simulink model "ALGO_Corner_Tanker_and_SP"  (Simulink 9.3)
settings: Solver=VariableStepAuto  StartTime=0  StopTime=15  RelTol=1e-3
libraries: simulink x22, Solver_SF x1
(part 2 of 2)

== matlab function 5DOF牵引车半挂车模型 50%液体 单摆模拟/TrailorTruck_5DOF_SP_50per ==
  data: vx input double; state output double; delta input double; observe output double
function [state,observe]=TrailorTruck_5DOF_SP(vx,delta)
%% 初始状态定义
%要记得设置本模块的采样时间哦
persistent Ts                             %采样时间    
persistent state0                         %上一时刻状态
if isempty(state0)
   Ts=0.01;%采样时间
   %初始化状态量
   vx10=vx(1);vx20=vx(2);
   vy10=0; df10=0;F10=0;dF10=0; Y10=0;X10=0;f10=0; %牵引车状态变量
   vy20=0; df20=0;F20=0;dF20=0; Y20=0;X20=-5.638315;f20=0;%半挂车状态变量
   th0=0; dth0=0;%等效摆状态变量
   state0=[vy10,df10,F10,dF10,vy20,df20,F20,dF20,...
       th0,dth0,f10,f20,vx10,vx20,Y10,X10,Y20,X20]';
   
end
%% 定义动力学模型参数
persistent a b c d e                    %轴距纵向几何参数
persistent Tw1 Tw2                      %轮距横向几何参数
persistent h1 h2 hc1 hc2                %质心至侧倾轴线距离
                                        %铰接点至侧倾轴线距离
persistent m1 m2 m1s m2s g;g=9.806;
persistent I1zz I1xx I1xz I2zz I2xx I2xz %惯性参量
persistent k1 k2 k3                      %线性轮胎模型参数
persistent kr1 kr2 c1 c2 k12             %悬架模型参数
persistent m0 mp h0 hp lp co             %等效摆模型参数
if isempty(a)
%摆模型参数
x=[10890,1.5,0.13,0.97,0.13];
sim_param=getParam_SP(x);
% sim_param=[m0,m1,h0+0.77,hp+0.77,lp,g,coeff];
m0=sim_param(1);
mp=sim_param(2);
h0=sim_param(3);
hp=sim_param(4);
lp=sim_param(5);
co=sim_param(7);
%车辆模型参数
L1=(5+6.27)/2;L2=(10.15+11.5)/2;       %轴距平均
a=1.385;b=L1-a;c=5.635-a;e=5.5;d=L2-e; %纵向几何
Tw1=(2.03+1.863*2)/3;Tw2=1.863;        %轮距平均
hm1s=1.02; %牵引车质心高度
hm2s=1.58; %50%充液率时半挂车质心高度
hhitch=1.1;%交接点高度
hroll1=0.2314;hroll2=0.9630;           %侧倾中心高度
h1=hm1s-hroll1;h2=hm2s-hroll2;hc1=hhitch-hroll1;hc2=hhitch-hroll2;%高度几何
m1s=6310;m1=m1s+570+785*2;             %牵引车质量
% m2s=5925;m2=m2s+665*2;               %半挂车空载质量
m2s=20387;m2=m2s+665*2;
I1xx=6879;I1xz=130;I1zz=19665;         %牵引车惯量
% I2xx=9960;I2xz=0;I2zz=179992;        %半挂车惯量
I2xx=9960;I2xz=0;I2zz=331380;
%轮胎模型参数
k1=-37e4;k2=-82e4;k3=-80e4;             %侧偏刚度
kr1=18.7e5;kr2=9.14e5;k12=68.3e5;       %侧倾刚度
c1=64.4e3;c2=197.7e3;                   %悬架等效阻尼
end
%% 定义线性动力学模型
dF2=state0(8);f1=state0(11);f2=state0(12);
vx1=vx(1);vx2=vx(2);
%线性车辆动力学模型
% M*dX = A0*X + B0*u
m14=-m1s*h1*c-I1xz;
m21=m1*vx1*hc1-m1s*h1*vx1;
m24=I1xx+2*m1s*h1^2-m1s*h1*hc1;
m55=m2*vx2*hc2-m2s*h2*vx2;
m58=I2xx+2*m2s*h2^2-m2s*h2*hc2;

M=[m1*vx1*c, I1zz, 0,   m14,     0,        0,   0,     0;
    m21,    -I1xz, 0,   m24,     0,        0,   0,     0;
   m1*vx1,      0, 0, -m1s*h1, m2*vx2,     0,   0, -m2s*h2;
     0,         0, 0,     0,  m2*vx2*e, -I2zz,  0, I2xz-m2s*h2*e;
     0,         0, 0,     0,    m55,    -I2xz,  0,    m58;
     1,    -c/vx1, 0, -hc1/vx1,  -1,   -e/vx2,  0, hc2/vx2;
     0,         0, 1,     0,     0,        0,   0,     0;
     0,         0, 0,     0,     0,        0,   1,     0   ];
 
 a11 = (c+a)*k1 + (c-b)*k2;
 a12 = a*(c+a)*k1/vx1 - b*(c-b)*k2/vx1 - m1*vx1*c;
 a22 = (a*k1-b*k2)*hc1/vx1 + (m1s*h1-m1*hc1)*vx1;
 a23 = m1s*g*h1 - kr1 -k12;
 a32 = (a*k1-b*k2)/vx1 - m1*vx1;
 a36 = -d*k3/vx2 - m2*vx2;
 a46 = -d*(e+d)*k3/vx2 - m2*vx2*e;
 a56 = (m2s*h2-m2*hc2)*vx2 - d*k3*hc2/vx2;
 a57 = m2s*g*h2 - kr2 -k12;
 %  X=   b1     df1    F1  dF1        b2  df2, F2   dF2 
 Acm0=[ a11,    a12,    0,   0,       0,   0,  0,    0;
   (k1+k2)*hc1, a22,  a23, -c1,       0,   0, k12,   0;
     k1+k2,     a32,    0,   0,      k3,  a36, 0,    0;
        0,       0,     0,   0, (e+d)*k3, a46, 0,    0;
        0,       0,    k12,  0,   k3*hc2, a56, a57, -c2;
        0,      -1,     0,   0,       0,   1,  0,    0;
        0,       0,     0,   1,       0,   0,  0,    0;
        0,       0,     0,   0,       0,   0,  0,    1   ];
    
 Bcm0=[-(c+a)*k1, -k1*hc1, -k1, 0, 0, 0, 0, 0]';
 

 %       1    2   3    4    5    6    7    8   9  10
%  X = vy1,  df1,F1, dF1, vy2, df2,  F2, dF2, th dth
% dX = dvy1;ddf1;dF1;ddF1;dvy2;ddf2;dF2;ddF2;dth;ddth ←M_
M_=zeros(10);
M_(9,9)=1;
M_(10,:)=[0,0,0,0,vx2/lp,0,0,hp/lp,0,1];
M_(3,:)=[0,0,0,0,(mp+m0)*vx2,0,(m0*h0+mp*(hp+lp))*dF2^2,-(m0+h0+mp*hp),0,mp*lp];
M_(4,:)=M_(3,:)*e;
M_(5,:)=M_(3,:)*hc2+...
[0,0,0,0,-(m0*h0+mp*hp)*vx2,0,0,(m0+h0^2+mp*hp^2),0,-mp*lp*hp];

A_=zeros(10);
A_(9,10)=1;
A_(10,:)=[0,0,0,0,0,-vx2/lp,0,0,-(hp/lp+1)*dF2^2-g/lp,-co];
A_(3,:)=[0,0,0,0,0,-(mp+m0)*vx2,0,0,0,0];
A_(4,:)=A_(3,:)*e;
A_(5,:)=A_(3,:)*hc2+...
[0,0,0,0,0,(m0*h0+mp*hp)*vx2,0,0,-mp*lp*g,0];
%       1    2   3    4    5    6    7    8   9  10
%  X =  0,   0,  0,   0,   0, df2,   0,   0, th  0
% dX =  0;   0;  0;   0;dvy2;   0;dF2;ddF2;dth;  0
 Acm=([M,zeros(8,2);zeros(2,10)]+M_)\([Acm0,zeros(8,2);zeros(2,10)]+A_);
 Bcm=([M,zeros(8,2);zeros(2,10)]+M_)\[Bcm0;zeros(2,1)];
 
 %% 增广状态量 并转变bi为vyi
 
 Trans=diag([vx1,1,1,1,vx2,1,1,1,1,1]);
 Ac=[Trans*Acm,zeros(10,8);            %增广状态量后的矩阵
     0,1,0,0,0,0,0,0,0,0,0,0,0,0,0,0,0,0;
     0,0,0,0,0,1,0,0,0,0,0,0,0,0,0,0,0,0;
     zeros(2,18);
     cos(f1),0,0,0,0,0,0,0,0,0,0,0,sin(f1),0,0,0,0,0;
    -sin(f1),0,0,0,0,0,0,0,0,0,0,0,cos(f1),0,0,0,0,0;
     0,0,0,0,cos(f2),0,0,0,0,0,0,0,0,sin(f2),0,0,0,0;
    0,0,0,0,-sin(f2),0,0,0,0,0,0,0,0,cos(f2),0,0,0,0  ];

 Bc=[Trans*Bcm;zeros(8,1)] ;
 
 %% 离散化线性模型
 [A,B]=c2d_zoh(Ac,Bc,Ts);             %离散化线性模型
 
%       1   2    3    4   5    6    7    8    9  10   11  12  13  14 15 16
% dX=[dvy1;ddf1;dF1;ddF1;dvy2;ddf2;dF2;ddF2;df1;df2;dvx1;dvx2;dY1;dX2;dY2;dX2];
%维度：14×1 

%% 更新状态量
%组装状态量
state=A*state0+B*delta;  %进行下一步更新
%% 观测量计算
%观测量为 Y1 X1 f1 th dth LTR1 LTR2
obsvMat=[zeros(2,14),eye(2),zeros(2,2); % Y1 X1
         zeros(1,10),1,zeros(1,7);      % f1
         zeros(2,8),eye(2),zeros(2,8);  % th dth
         2/(Tw1*m1*g)*[0,0,-(kr1+k12),-c1,0,0,k12,0],zeros(1,10);%LTR1
         2/(Tw2*m2*g)*[0,0,k12,0,0,0,-(kr2+k12),-c2],zeros(1,10);%LTR2
         ];
observe=obsvMat*state;
%% 拆解状态量并为下一步计算保存

state0=state;



end
%% 根据变量获取参数
function sim_param=getParam_SP(x)
%根据变量生成传输参数
TotMass=14462;
m1=x(1);%参数1
m0=TotMass-m1;
h0=x(2);%参数2
hp=x(3);%参数3
lp=x(4);%参数4
g=9.806;
coeff=x(5);%参数5
sim_param=[m0,m1,h0+0.77,hp+0.77,lp,g,coeff];
end
